simulink model "q_heli3d_semestral_project"  (Simulink 8.9)
settings: Solver=ode1  StartTime=0.0  StopTime=inf  FixedStep=0.002  RelTol=1e-3  EnableMultiTasking=on
values from neighbouring files (symbols this model uses):
  ae1 = model_identified_MF1.Parameters(3).Value    [model_benchmark_init.m]    (also in workspace.mat = 1.36231449822)
  ae2 = model_identified_MF1.Parameters(4).Value    [model_benchmark_init.m]    (also in workspace.mat = -0.378717172069)
  at = model_identified_MF1.Parameters(7).Value    [model_benchmark_init.m]    (also in workspace.mat = -0.463804529993)
  be = model_identified_MF1.Parameters(6).Value    [model_benchmark_init.m]    (also in workspace.mat = 0.116311837295)
  bl = model_identified_MF1.Parameters(2).Value    [model_benchmark_init.m]    (also in workspace.mat = 0.103160863637)
  bt = model_identified_MF1.Parameters(9).Value    [model_benchmark_init.m]    (also in workspace.mat = 0.962119048974)
  ce = model_identified_MF1.Parameters(5).Value    [model_benchmark_init.m]    (also in workspace.mat = 0.04469700002)
  cl = model_identified_MF1.Parameters(1).Value    [model_benchmark_init.m]    (also in workspace.mat = 0.202457747385)
  ct = model_identified_MF1.Parameters(8).Value    [model_benchmark_init.m]    (also in workspace.mat = 0.00762763482449)
  elev_0 = -0.479965544298    [workspace.mat]
  K_AMP = 3    [workspace.mat]
  K_EC_E = -0.00153398078789    [workspace.mat]
  K_EC_P = 0.00153398078789    [workspace.mat]
  K_EC_T = 0.000766990393943    [workspace.mat]
  VMAX_AMP = 24    [workspace.mat]
  VMAX_DAC = 10    [workspace.mat]
  wcf = 125.663706144    [workspace.mat]
  x0 = [0; 0; 0; 0; 0; 0]    [model_benchmark_init.m]    (also in model_benchmark_ode45.m = [0; 0; 0; 0; 0.1; 0]; workspace.mat = [0 0 0.1745 0 -0.1047 0])
  zetaf = 0.9    [workspace.mat]
undefined symbols (not defined in the file or in its folder): HIL, qc_get_step_size
libraries: quarc_library x4, simulink_extras x1
settings Model: Creator=MLevis  LastModifiedBy=obrusvit  SimulationMode=external  ExtModeTrigDuration=100000
settings SolverCC: PositivePriorityOrder=on
settings DataIOCC: LimitDataPoints=off
settings OptimizationCC: ExpressionDepthLimit=2147483647  InitFltsAndDblsToZero=on
settings DebuggingCC: SaveWithParameterizedLinksMsg=none  SolverPrmCheckMsg=warning
settings RTWCC: SystemTargetFile=quarc_win64.tlc  TemplateMakefile=quarc_default_tmf  Description=QUARC Win64 Target
settings STFCustomTargetCC: TargetPreCompLibLocation=C:\PROGRA~3\QUARC\lib\2017a\win64\release  ConcurrentExecutionCompliant=on  GeneratePreprocessorConditionals=Disable all  SystemTargetFile=quarc_win64.tlc
settings GRTTargetCC: TargetPreCompLibLocation=C:\PROGRA~3\QUARC\lib\2017a\win64\release  ParMdlRefBuildCompliant=off  CompOptLevelCompliant=off  MatFileLogging=off  CPPClassGenCompliant=off  UseToolchainInfoCompliant=off  ExtMode=on  ExtModeMexFile=quarc_comm

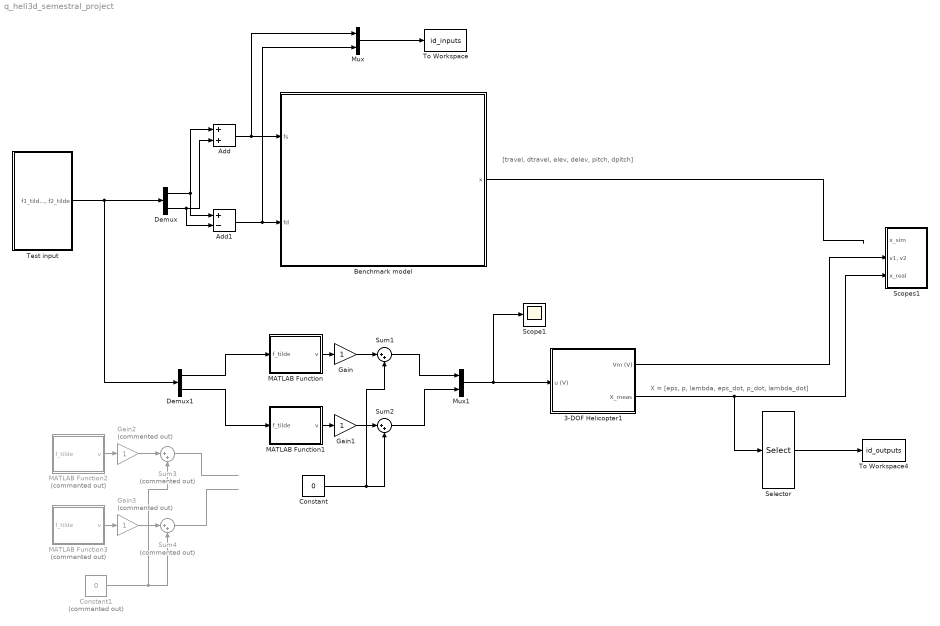
== system q_heli3d_semestral_project ==
  note: X = [eps, p, lambda, eps_dot, p_dot, lambda_dot]
  note: [travel, dtravel, elev, delev, pitch, dpitch]
  3-DOF Helicopter1 : Subsystem
  Add : Sum
  Add1 : Sum  Inputs=+-
  Benchmark model : Subsystem
  Constant : Constant  Value=0
  Constant1 : Constant  Commented=on  Value=0
  Demux : Demux  Outputs=2
  Demux1 : Demux  Outputs=2
  Gain : Gain
  Gain1 : Gain
  Gain2 : Gain  Commented=on
  Gain3 : Gain  Commented=on
  MATLAB Function : MATLAB Function  TreatAsAtomicUnit=on
  MATLAB Function1 : MATLAB Function  TreatAsAtomicUnit=on
  MATLAB Function2 : MATLAB Function  Commented=on  TreatAsAtomicUnit=on
  MATLAB Function3 : MATLAB Function  Commented=on  TreatAsAtomicUnit=on
  Mux : Mux  Inputs=2
  Mux1 : Mux  Inputs=2
  Scope1 : Scope
  Scopes1 : Subsystem
  Selector : Selector  InputPortWidth=6  IndexOptions=Index vector (dialog)  Indices=[3 1 2]  OutputSizes=1
  Sum1 : Sum  Inputs=|++
  Sum2 : Sum  Inputs=|++
  Sum3 : Sum  Commented=on  Inputs=|++
  Sum4 : Sum  Commented=on  Inputs=|++
  Test input : Subsystem
  To Workspace : ToWorkspace  VariableName=id_inputs  SampleTime=0.002
  To Workspace4 : ToWorkspace  VariableName=id_outputs  SampleTime=0.002
  wires:
  Test input/1("f1_tilde, f2_tilde") -> Demux1/1, Demux/1
  Mux1/1 -> 3-DOF Helicopter1/1(u (V)), Scope1/1
  Add1/1 -> Mux/2, Benchmark model/2("fd ")
  Benchmark model/1(x) -> ?
  Add/1 -> Mux/1, Benchmark model/1("fs ")
  Demux/1 -> Add1/1, Add/1
  Demux/2 -> Add1/2, Add/2
  3-DOF Helicopter1/2(X_meas) -> Selector/1, Scopes1/3(x_real)
  3-DOF Helicopter1/1(Vm (V)) -> Scopes1/2("v1, v2 ")
  Mux/1 -> To Workspace/1
  Selector/1 -> To Workspace4/1
  Gain3/1 -> Sum4/1
  Sum4/1 -> ?
  Constant1/1 -> Sum3/2, Sum4/2
  MATLAB Function2/1(v) -> Gain2/1
  MATLAB Function3/1(v) -> Gain3/1
  Gain2/1 -> Sum3/1
  ? -> MATLAB Function3/1(f_tilde)
  Sum3/1 -> ?
  ? -> MATLAB Function2/1(f_tilde)
  Gain1/1 -> Sum2/1
  Sum2/1 -> Mux1/2
  Constant/1 -> Sum1/2, Sum2/2
  MATLAB Function/1(v) -> Gain/1
  MATLAB Function1/1(v) -> Gain1/1
  Gain/1 -> Sum1/1
  Demux1/2 -> MATLAB Function1/1(f_tilde)
  Sum1/1 -> Mux1/1
  Demux1/1 -> MATLAB Function/1(f_tilde)

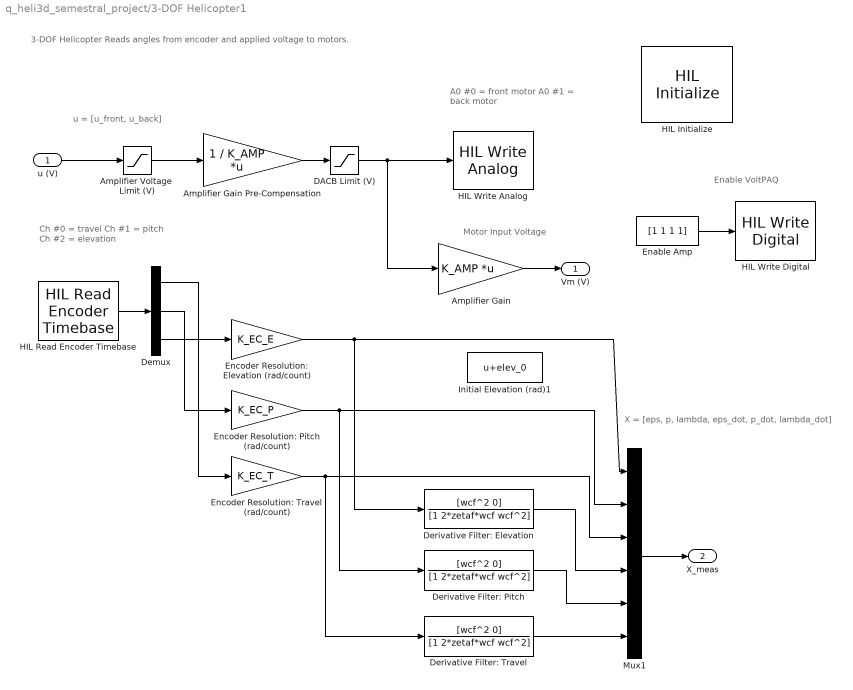
== system q_heli3d_semestral_project/3-DOF Helicopter1 ==
  note: Enable VoltPAQ
  note: X = [eps, p, lambda, eps_dot, p_dot, lambda_dot]
  note: Ch #0 = travel
      | Ch #1 = pitch
      | Ch #2 = elevation
  note: 3-DOF Helicopter
      | Reads angles from encoder and applied voltage to motors.
  note: Motor Input Voltage
  note: u = [u_front, u_back]
  note: A0 #0 = front motor
      | A0 #1 = back motor
  u (V) : Inport
  Amplifier Gain : Gain  Gain=K_AMP  Multiplication=Matrix(K*u)  SaturateOnIntegerOverflow=on  OutDataTypeStr=Inherit: Same as input  ParamDataTypeStr=Inherit: Same as input
  Amplifier Gain Pre-Compensation : Gain  Gain=1 / K_AMP  Multiplication=Matrix(K*u)  SaturateOnIntegerOverflow=on  OutDataTypeStr=Inherit: Same as input  ParamDataTypeStr=Inherit: Same as input
  Amplifier Voltage  Limit (V) : Saturate  UpperLimit=VMAX_AMP  LowerLimit=-VMAX_AMP
  DACB Limit (V) : Saturate  UpperLimit=VMAX_DAC  LowerLimit=-VMAX_DAC
  Demux : Demux  Outputs=3
  Derivative Filter: Elevation : TransferFcn  Numerator=[wcf^2 0]  Denominator=[1 2*zetaf*wcf wcf^2]
  Derivative Filter: Pitch : TransferFcn  Numerator=[wcf^2 0]  Denominator=[1 2*zetaf*wcf wcf^2]
  Derivative Filter: Travel : TransferFcn  Numerator=[wcf^2 0]  Denominator=[1 2*zetaf*wcf wcf^2]
  Enable Amp : Constant  Value=[1 1 1 1]
  Encoder Resolution: Elevation (rad/count) : Gain  Gain=K_EC_E
  Encoder Resolution: Pitch (rad/count) : Gain  Gain=K_EC_P
  Encoder Resolution: Travel (rad/count) : Gain  Gain=K_EC_T
  HIL Initialize : quarc_library/Data Acquisition/Generic/Configuration/HIL Initialize  object_name=HIL-1  board_type=q8_usb  board_number=0  board_options=update_rate=normal;decimation=1  exclusive=off  active=on  hardware_clocks=[0:2]  clock_modes=[]  initial_clock_frequencies=[]  set_clock_params_at_start=off  set_clock_params_at_switch_in=off  set_clock_frequencies_at_start=off  set_clock_frequencies_at_switch_in=off  analog_input_channels=[0:7]  analog_input_configurations=[]  analog_input_maximums=10  analog_input_minimums=-10  set_analog_input_params_at_start=on  set_analog_input_params_at_switch_in=off  analog_output_channels=[0:7]  analog_output_maximums=10  analog_output_minimums=-10  initial_analog_outputs=[0]  final_analog_outputs=[0]  watchdog_analog_outputs=0  set_analog_output_params_at_start=on  set_analog_output_params_at_switch_in=off  set_analog_outputs_at_start=on  set_analog_outputs_at_switch_in=off  set_analog_outputs_at_terminate=on  set_analog_outputs_at_switch_out=off  set_analog_outputs_on_watchdog=off  digital_input_channels=[]  digital_output_channels=[]  digital_output_configuration=[]  initial_digital_outputs=[1]  final_digital_outputs=[1]  watchdog_digital_outputs=[1]  set_digital_output_params_at_start=off  set_digital_output_params_at_switch_in=off  set_digital_outputs_at_start=on  set_digital_outputs_at_switch_in=off  set_digital_outputs_at_terminate=on  set_digital_outputs_at_switch_out=off  set_digital_outputs_on_watchdog=off  encoder_channels=[0:7]  quadrature=[4]  encoder_filter_frequency=[]  initial_encoder_counts=[0]  set_encoder_params_at_start=on  set_encoder_params_at_switch_in=off  set_encoder_counts_at_start=on  set_encoder_counts_at_switch_in=off  pwm_channels=[0:7]  pwm_modes=0  pwm_frequency=99.532799999999995e6/4095  pwm_configuration=[0]  pwm_alignment=[0]  pwm_polarity=[1]  pwm_leading_deadband=[0]  pwm_trailing_deadband=[0]  initial_pwm_outputs=[0]  final_pwm_outputs=[0]  watchdog_pwm_outputs=[0]  set_pwm_params_at_start=on  set_pwm_params_at_switch_in=off  set_pwm_outputs_at_start=on  set_pwm_outputs_at_switch_in=off  set_pwm_outputs_at_terminate=on  set_pwm_outputs_at_switch_out=off  set_pwm_outputs_on_watchdog=off  other_output_channels=[]  initial_other_outputs=[]  final_other_outputs=[]  watchdog_other_outputs=[]  set_other_outputs_at_start=off  set_other_outputs_at_switch_in=off  set_other_outputs_at_terminate=off  set_other_outputs_at_switch_out=off  set_other_outputs_on_watchdog=off
  HIL Read Encoder Timebase : quarc_library/Data Acquisition/Generic/Timebases/HIL Read Encoder Timebase  object_name=HIL-1  clock=0  channels=[0:2]  samples_in_buffer=max(ceil(1/qc_get_step_size), 1)  active=on  vector_output=on  data_type_mode=Inherit via back propagation  data_type=double
  HIL Write Analog : quarc_library/Data Acquisition/Generic/Immediate I//O/HIL Write Analog  object_name=HIL-1  channels=[0,1]  sample_time=-1  active=off  vector_input=on
  HIL Write Digital : quarc_library/Data Acquisition/Generic/Immediate I//O/HIL Write Digital  object_name=HIL-1  channels=[0:3]  sample_time=-1  active=off  vector_input=on
      settings: SourceProductName=QUARC Targets
  Initial Elevation (rad)1 : Bias  Bias=elev_0
  Mux1 : Mux  Inputs=6
  Vm (V) : Outport
  X_meas : Outport  Port=2
  wires:
  Enable Amp/1 -> HIL Write Digital/1
  Encoder Resolution: Elevation (rad/count)/1 -> Mux1/1, Derivative Filter: Elevation/1
  Derivative Filter: Travel/1 -> Mux1/6
  Derivative Filter: Pitch/1 -> Mux1/5
  Derivative Filter: Elevation/1 -> Mux1/4
  Encoder Resolution: Travel (rad/count)/1 -> Derivative Filter: Travel/1, Mux1/3
  Encoder Resolution: Pitch (rad/count)/1 -> Derivative Filter: Pitch/1, Mux1/2
  Demux/2 -> Encoder Resolution: Pitch (rad/count)/1
  Demux/1 -> Encoder Resolution: Travel (rad/count)/1
  Demux/3 -> Encoder Resolution: Elevation (rad/count)/1
  DACB Limit (V)/1 -> HIL Write Analog/1, Amplifier Gain/1
  u (V)/1 -> Amplifier Voltage  Limit (V)/1
  Amplifier Gain/1 -> Vm (V)/1
  Amplifier Voltage  Limit (V)/1 -> Amplifier Gain Pre-Compensation/1
  Amplifier Gain Pre-Compensation/1 -> DACB Limit (V)/1
  Mux1/1 -> X_meas/1
  HIL Read Encoder Timebase/1 -> Demux/1

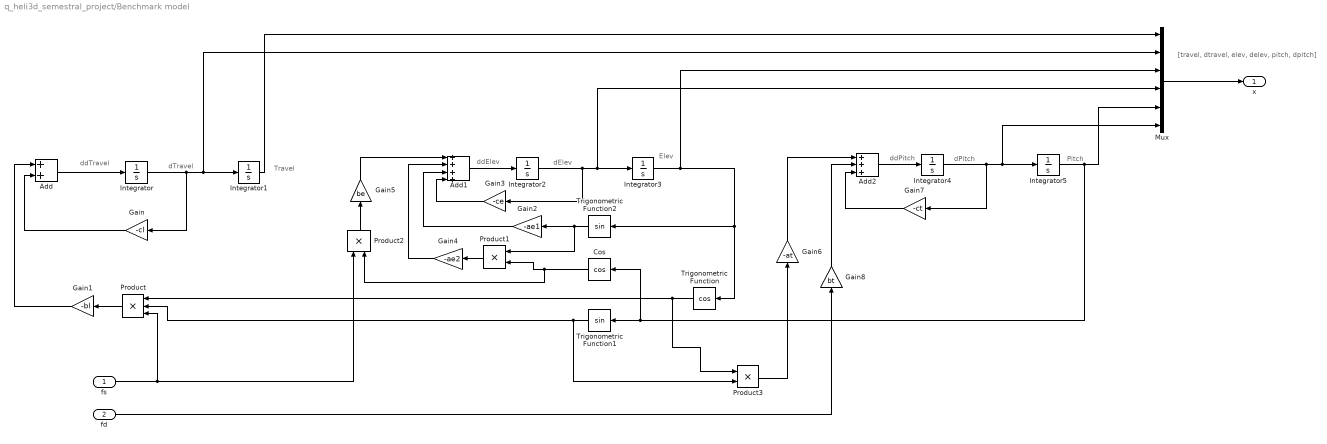
== system q_heli3d_semestral_project/Benchmark model ==
  note: [travel, dtravel, elev, delev, pitch, dpitch]
  note: Pitch
  note: dPitch
  note: ddPitch
  note: Elev
  note: dElev
  note: ddElev
  note: Travel
  note: dTravel
  note: ddTravel
  "fs " : Inport
  "fd " : Inport  Port=2
  Add : Sum
  Add1 : Sum  Inputs=++++
  Add2 : Sum  Inputs=+++
  Cos : Trigonometry  Operator=cos
  Gain : Gain  Gain=-cl
  Gain1 : Gain  Gain=-bl
  Gain2 : Gain  Gain=-ae1
  Gain3 : Gain  Gain=-ce
  Gain4 : Gain  Gain=-ae2
  Gain5 : Gain  Gain=be
  Gain6 : Gain  Gain=-at
  Gain7 : Gain  Gain=-ct
  Gain8 : Gain  Gain=bt
  Integrator : Integrator  InitialCondition=x0(2)
  Integrator1 : Integrator  InitialCondition=x0(1)
  Integrator2 : Integrator  InitialCondition=x0(4)
  Integrator3 : Integrator
  Integrator4 : Integrator  InitialCondition=x0(6)
  Integrator5 : Integrator  InitialCondition=x0(5)
  Mux : Mux  Inputs=6
  Product : Product  Inputs=3
  Product1 : Product
  Product2 : Product
  Product3 : Product
  Trigonometric Function : Trigonometry  Operator=cos
  Trigonometric Function1 : Trigonometry
  Trigonometric Function2 : Trigonometry
  x : Outport
  wires:
  Gain5/1 -> Add1/1
  Product/1 -> Gain1/1
  Product2/1 -> Gain5/1
  "fd "/1 -> Gain8/1
  Trigonometric Function/1 -> Product3/1, Product/1
  Gain7/1 -> Add2/3
  Cos/1 -> Product2/2, Product1/2
  Gain4/1 -> Add1/2
  Gain2/1 -> Add1/3
  Mux/1 -> x/1
  Gain8/1 -> Add2/2
  Add2/1 -> Integrator4/1
  Gain6/1 -> Add2/1
  Integrator1/1 -> Mux/1
  Gain1/1 -> Add/1
  Integrator3/1 -> Mux/3, Trigonometric Function2/1, Trigonometric Function/1
  Integrator2/1 -> Gain3/1, Mux/4, Integrator3/1
  Product1/1 -> Gain4/1
  Gain3/1 -> Add1/4
  Integrator4/1 -> Gain7/1, Mux/6, Integrator5/1
  Integrator/1 -> Gain/1, Integrator1/1, Mux/2
  Gain/1 -> Add/2
  Add1/1 -> Integrator2/1
  Integrator5/1 -> Cos/1, Trigonometric Function1/1, Mux/5
  Trigonometric Function2/1 -> Product1/1, Gain2/1
  Trigonometric Function1/1 -> Product3/2, Product/2
  "fs "/1 -> Product2/1, Product/3
  Add/1 -> Integrator/1
  Product3/1 -> Gain6/1

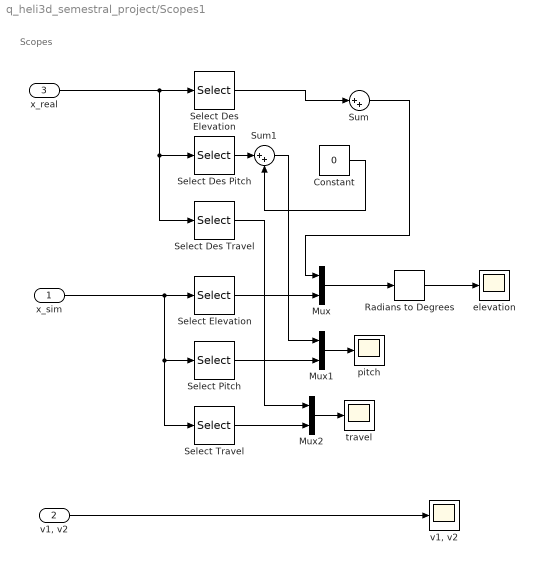
== system q_heli3d_semestral_project/Scopes1 ==
  note: Scopes
  x_sim : Inport
  "v1, v2 " : Inport  Port=2
  x_real : Inport  Port=3
  Constant : Constant  Value=0
  Mux : Mux  Inputs=2
  Mux1 : Mux  Inputs=2
  Mux2 : Mux  Inputs=2
  Radians to Degrees : simulink_extras/Transformations/Radians to Degrees
  Select Des Elevation : Selector  InputPortWidth=6  IndexOptions=Index vector (dialog)  Indices=1  OutputSizes=1
  Select Des Pitch : Selector  InputPortWidth=6  IndexOptions=Index vector (dialog)  Indices=2  OutputSizes=1
  Select Des Travel : Selector  InputPortWidth=6  IndexOptions=Index vector (dialog)  Indices=3  OutputSizes=1
  Select Elevation : Selector  InputPortWidth=6  IndexOptions=Index vector (dialog)  Indices=3  OutputSizes=1
  Select Pitch : Selector  InputPortWidth=6  IndexOptions=Index vector (dialog)  Indices=5  OutputSizes=1
  Select Travel : Selector  InputPortWidth=6  IndexOptions=Index vector (dialog)  Indices=1  OutputSizes=1
  Sum : Sum  Inputs=|++
  Sum1 : Sum  Inputs=|++
  "elevation " : Scope
  pitch : Scope
  travel : Scope
  "v1, v2" : Scope
  wires:
  Mux/1 -> Radians to Degrees/1
  Mux1/1 -> pitch/1
  "v1, v2 "/1 -> "v1, v2"/1
  Mux2/1 -> travel/1
  Select Elevation/1 -> Mux/2
  Select Pitch/1 -> Mux1/2
  Select Travel/1 -> Mux2/2
  Select Des Elevation/1 -> Sum/1
  Select Des Pitch/1 -> Sum1/1
  Select Des Travel/1 -> Mux2/1
  x_sim/1 -> Select Elevation/1, Select Pitch/1, Select Travel/1
  x_real/1 -> Select Des Elevation/1, Select Des Pitch/1, Select Des Travel/1
  Sum/1 -> Mux/1
  Constant/1 -> Sum1/2
  Sum1/1 -> Mux1/1
  Radians to Degrees/1 -> "elevation "/1

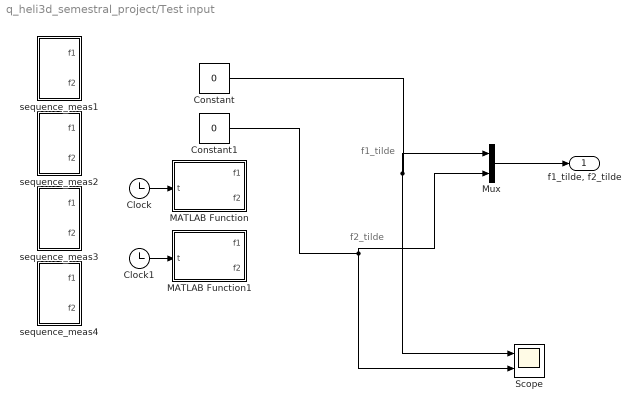
== system q_heli3d_semestral_project/Test input ==
  note: f2_tilde
  note: f1_tilde
  Clock : Clock
  Clock1 : Clock
  Constant : Constant  Value=0
  Constant1 : Constant  Value=0
  MATLAB Function : MATLAB Function  TreatAsAtomicUnit=on
  MATLAB Function1 : MATLAB Function  TreatAsAtomicUnit=on
  Mux : Mux  Inputs=2
  Scope : Scope  NumInputPorts=2
  sequence_meas1 : Subsystem
  sequence_meas2 : Subsystem
  sequence_meas3 : Subsystem
  sequence_meas4 : Subsystem
  "f1_tilde, f2_tilde" : Outport
  wires:
  Mux/1 -> "f1_tilde, f2_tilde"/1
  Constant/1 -> Mux/1, Scope/1
  Constant1/1 -> Scope/2, Mux/2
  Clock/1 -> MATLAB Function/1(t)
  Clock1/1 -> MATLAB Function1/1(t)

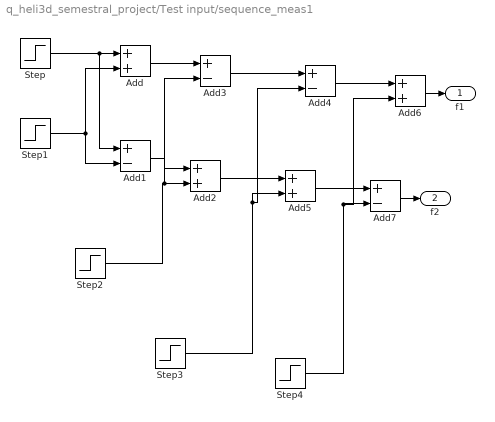
== system q_heli3d_semestral_project/Test input/sequence_meas1 ==
  Add{,2,5..6} (4 alike) : Sum
  Add{1,3..4,7} (4 alike) : Sum  Inputs=+-
  Step : Step  Time=5  After=0.6  SampleTime=0
  Step1 : Step  Time=10  After=0.2  SampleTime=0
  Step2 : Step  Time=11  After=0.2  SampleTime=0
  Step3 : Step  Time=11  After=0.4  SampleTime=0
  Step4 : Step  Time=14.2  After=0.4  SampleTime=0
  f1 : Outport
  "f2 " : Outport  Port=2
  wires:
  Add5/1 -> Add7/1
  Step2/1 -> Add3/2, Add2/2
  Step3/1 -> Add4/2, Add5/2
  Add1/1 -> Add2/1
  Add3/1 -> Add4/1
  Step/1 -> Add1/1, Add/1
  Step1/1 -> Add/2, Add1/2
  Add4/1 -> Add6/1
  Add/1 -> Add3/1
  Add2/1 -> Add5/1
  Step4/1 -> Add6/2, Add7/2
  Add6/1 -> f1/1
  Add7/1 -> "f2 "/1

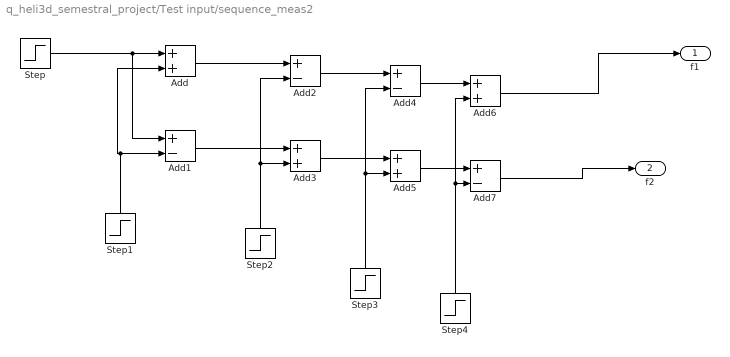
== system q_heli3d_semestral_project/Test input/sequence_meas2 ==
  Add{,3,5..6} (4 alike) : Sum
  Add{1..2,4,7} (4 alike) : Sum  Inputs=+-
  Step : Step  Time=5  After=0.4  SampleTime=0
  Step1 : Step  Time=10  After=0.3  SampleTime=0
  Step2 : Step  Time=11  After=0.3  SampleTime=0
  Step3 : Step  Time=11  After=0.6  SampleTime=0
  Step4 : Step  Time=12.5  After=0.6  SampleTime=0
  f1 : Outport
  "f2 " : Outport  Port=2
  wires:
  Add7/1 -> "f2 "/1
  Add6/1 -> f1/1
  Add5/1 -> Add7/1
  Add1/1 -> Add3/1
  Add/1 -> Add2/1
  Add3/1 -> Add5/1
  Step2/1 -> Add3/2, Add2/2
  Step4/1 -> Add6/2, Add7/2
  Add2/1 -> Add4/1
  Step1/1 -> Add/2, Add1/2
  Add4/1 -> Add6/1
  Step/1 -> Add1/1, Add/1
  Step3/1 -> Add4/2, Add5/2

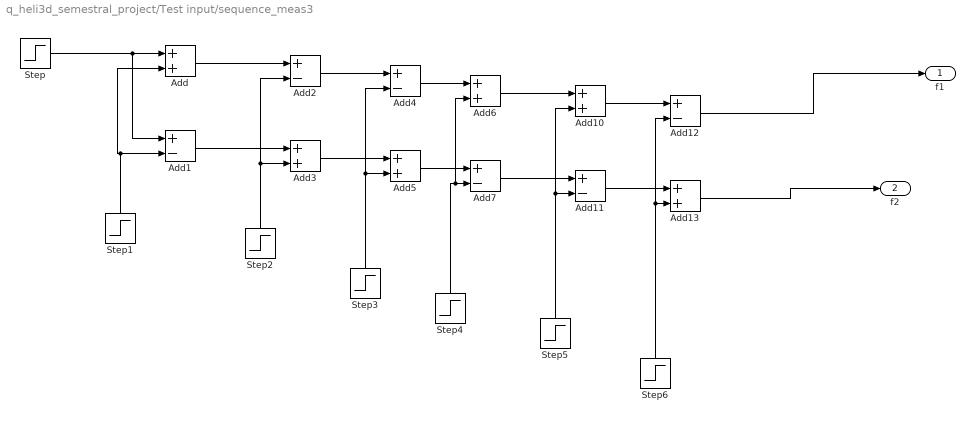
== system q_heli3d_semestral_project/Test input/sequence_meas3 ==
  Add{,3,5..6,10,13} (6 alike) : Sum
  Add{1..2,4,7,11..12} (6 alike) : Sum  Inputs=+-
  Step : Step  Time=2  After=0.2  SampleTime=0
  Step1 : Step  Time=4  After=0.1  SampleTime=0
  Step2 : Step  Time=6.5  After=0.1  SampleTime=0
  Step3 : Step  Time=6.5  After=0.5  SampleTime=0
  Step4 : Step  Time=9.8  After=0.5  SampleTime=0
  Step5 : Step  Time=9.8  After=0.5  SampleTime=0
  Step6 : Step  Time=12  After=0.5  SampleTime=0
  f1 : Outport
  "f2 " : Outport  Port=2
  wires:
  Add13/1 -> "f2 "/1
  Add12/1 -> f1/1
  Step/1 -> Add1/1, Add/1
  Add5/1 -> Add7/1
  Add4/1 -> Add6/1
  Add6/1 -> Add10/1
  Step4/1 -> Add6/2, Add7/2
  Add3/1 -> Add5/1
  Step1/1 -> Add/2, Add1/2
  Add/1 -> Add2/1
  Step2/1 -> Add3/2, Add2/2
  Add11/1 -> Add13/1
  Add1/1 -> Add3/1
  Add10/1 -> Add12/1
  Step6/1 -> Add13/2, Add12/2
  Add7/1 -> Add11/1
  Step5/1 -> Add11/2, Add10/2
  Add2/1 -> Add4/1
  Step3/1 -> Add4/2, Add5/2

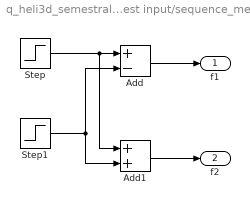
== system q_heli3d_semestral_project/Test input/sequence_meas4 ==
  Add : Sum  Inputs=+-
  Add1 : Sum
  Step : Step  Time=5  After=0.2  SampleTime=0
  Step1 : Step  Time=10  After=0.03  SampleTime=0
  f1 : Outport
  "f2 " : Outport  Port=2
  wires:
  Add/1 -> f1/1
  Add1/1 -> "f2 "/1
  Step1/1 -> Add/2, Add1/2
  Step/1 -> Add1/1, Add/1

== matlab function MATLAB Function1 ==
  data: f_tilde input double; v output double
function v = fcn(f_tilde)

v = scaled_force_2_voltage_new(f_tilde);

== matlab function MATLAB Function ==
  data: f_tilde input double; v output double
function v = fcn(f_tilde)

v = scaled_force_2_voltage_new(f_tilde);

== matlab function Test input/MATLAB Function ==
  data: t input double; f1 output double; f2 output double
function [f1,f2] = fcn(t)

if t <= 5
    f1 = 0;
    f2 = 0;
elseif t <= 15
    f1 = 0.4;
    f2 = 0.4;
else
    f1 = 0;
    f2 = 0;
end

== matlab function MATLAB Function2 ==
  data: f_tilde input double; v output double; par_inputs parameter double
function v = fcn(f_tilde, par_inputs)

v = scaled_force_2_voltage(f_tilde, par_inputs.scaled_f_2_v_par, par_inputs.scaled_f_2_v_ths);

== matlab function Test input/MATLAB Function1 ==
  data: t input double; f1 output double; f2 output double
function [f1,f2] = fcn(t)

if t <= 2
    f1 = 0;
    f2 = 0;
elseif t <= 8
    f1 = 0.5;
    f2 = 0.5;
elseif t <= 10
    f1 = 0.6;
    f2 = 0.4;
elseif t <= 12
    f1 = 0.3;
    f2 = 0.7;
else
    f1 = 0;
    f2 = 0;
end

== matlab function MATLAB Function3 ==
  data: f_tilde input double; v output double; par_inputs parameter double
function v = fcn(f_tilde, par_inputs)

v = scaled_force_2_voltage(f_tilde, par_inputs.scaled_f_2_v_par, par_inputs.scaled_f_2_v_ths);
